simulink library "EBCAN"  (R2017a)
settings: Solver=VariableStepAuto  StartTime=0.0  StopTime=10.0  RelTol=1e-3
settings Model: Creator=Di Russo  LastModifiedBy=Vraj M

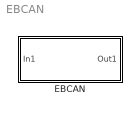
== system EBCAN ==
  EBCAN : Subsystem

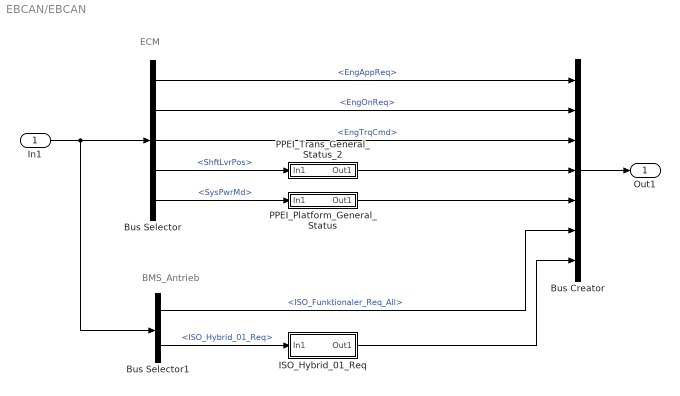
== system EBCAN/EBCAN ==
  note: ECM
  note: BMS_Antrieb
  In1 : Inport
  Bus Creator : BusCreator  Inputs=7
  Bus Selector : BusSelector  OutputSignals=Controls.EngAppReq,Controls.EngOnReq,Controls.EngTrqCmd,Controls.ShftLvrPos,Controls.SysPwrMd
  Bus Selector1 : BusSelector  OutputSignals=BMS_CAN.ISO_Funktionaler_Req_All,BMS_CAN.ISO_Hybrid_01_Req
  ISO_Hybrid_01_Req : Subsystem
  PPEI_Platform_General_Status : Subsystem
  PPEI_Trans_General_Status_2 : Subsystem
  Out1 : Outport
  wires:
  Bus Selector1/2 -> ISO_Hybrid_01_Req/1(In1)  "<ISO_Hybrid_01_Req>"
  ISO_Hybrid_01_Req/1(Out1) -> Bus Creator/7
  In1/1 -> Bus Selector/1, Bus Selector1/1
  Bus Selector1/1 -> Bus Creator/6  "<ISO_Funktionaler_Req_All>"
  Bus Selector/1 -> Bus Creator/1  "<EngAppReq>"
  Bus Selector/2 -> Bus Creator/2  "<EngOnReq>"
  Bus Selector/3 -> Bus Creator/3  "<EngTrqCmd>"
  PPEI_Trans_General_Status_2/1(Out1) -> Bus Creator/4
  Bus Selector/5 -> PPEI_Platform_General_Status/1(In1)  "<SysPwrMd>"
  Bus Selector/4 -> PPEI_Trans_General_Status_2/1(In1)  "<ShftLvrPos>"
  PPEI_Platform_General_Status/1(Out1) -> Bus Creator/5
  Bus Creator/1 -> Out1/1

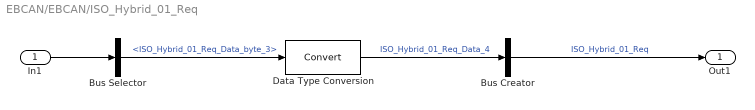
== system EBCAN/EBCAN/ISO_Hybrid_01_Req ==
  In1 : Inport
  Bus Creator : BusCreator  Inputs=1
  Bus Selector : BusSelector  OutputSignals=ISO_Hybrid_01_Req_Data_byte_3
  Data Type Conversion : DataTypeConversion
  Out1 : Outport
  wires:
  Bus Selector/1 -> Data Type Conversion/1  "<ISO_Hybrid_01_Req_Data_byte_3>"
  Bus Creator/1 -> Out1/1  "ISO_Hybrid_01_Req"
  Data Type Conversion/1 -> Bus Creator/1  "ISO_Hybrid_01_Req_Data_4"
  In1/1 -> Bus Selector/1

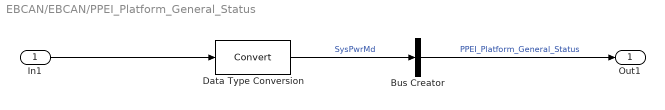
== system EBCAN/EBCAN/PPEI_Platform_General_Status ==
  In1 : Inport
  Bus Creator : BusCreator  Inputs=1
  Data Type Conversion : DataTypeConversion
  Out1 : Outport
  wires:
  In1/1 -> Data Type Conversion/1
  Data Type Conversion/1 -> Bus Creator/1  "SysPwrMd"
  Bus Creator/1 -> Out1/1  "PPEI_Platform_General_Status"

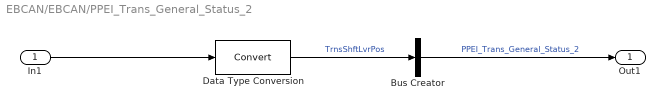
== system EBCAN/EBCAN/PPEI_Trans_General_Status_2 ==
  In1 : Inport
  Bus Creator : BusCreator  Inputs=1
  Data Type Conversion : DataTypeConversion
  Out1 : Outport
  wires:
  Bus Creator/1 -> Out1/1  "PPEI_Trans_General_Status_2"
  Data Type Conversion/1 -> Bus Creator/1  "TrnsShftLvrPos"
  In1/1 -> Data Type Conversion/1
